simulink model "PNG3"  (R2021b)
settings: Solver=VariableStepAuto  StartTime=0.0  StopTime=45  RelTol=1e-3
values from neighbouring files (symbols this model uses):
  d2r = pi/180    (= 0.0174532925199)    [PN_Guidance_matlab.m]
  Ka = 4.5    [PN_Guidance_matlab.m]
  Kdc = 1.12    [PN_Guidance_matlab.m]
  Ki = 14.3    [PN_Guidance_matlab.m]
  Kr = -0.37    [PN_Guidance_matlab.m]
  l_M0 = 80*d2r    (= 1.3962634016)    [PN_Guidance_matlab.m]
  l_T0 = -2.5*d2r    (= -0.0436332312999)    [PN_Guidance_matlab.m]
  V_T = 600    [PN_Guidance_matlab.m]
  X_M0 = 2000    [PN_Guidance_matlab.m]
  X_T0 = 100    [PN_Guidance_matlab.m]
  Z_M0 = 0    [PN_Guidance_matlab.m]
  Z_T0 = 20000    [PN_Guidance_matlab.m]
libraries: simulink x1
settings Model: Creator=rocke  LastModifiedBy=rocke
settings SolverCC: ZeroCrossAlgorithm=Adaptive
settings DebuggingCC: IgnoredZcDiagnostic=none
settings SFSimCC: LegacyBehaviorForPersistentVarInContinuousTime=on

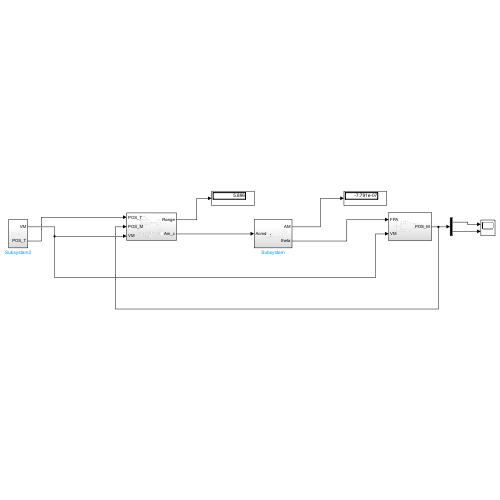
[thumbnail: Simulink's stored preview of the top-level diagram]
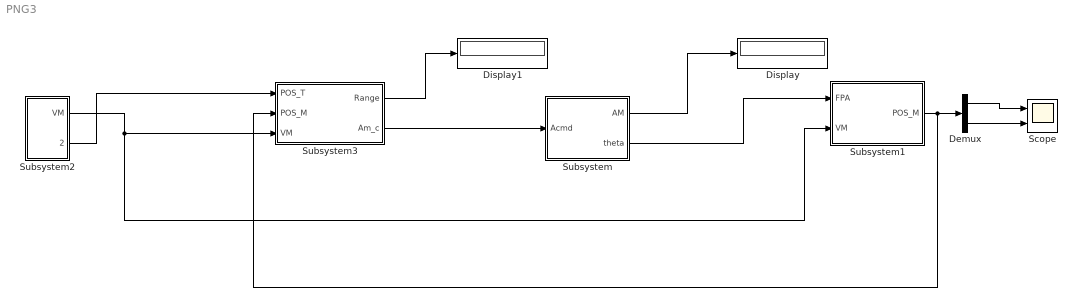
== system PNG3 ==
  Demux : Demux  Outputs=2
  Display : Display
  Display1 : Display
  Scope : Scope  NumInputPorts=2
  Subsystem : Subsystem
  Subsystem1 : Subsystem
  Subsystem2 : Subsystem
  Subsystem3 : Subsystem
  wires:
  Subsystem1/1(POS_M) -> Subsystem3/2(POS_M), Demux/1
  Demux/1 -> Scope/1
  Subsystem2/1(VM) -> Subsystem3/3(VM), Subsystem1/2(VM)
  Subsystem2/2(POS_T) -> Subsystem3/1(POS_T)
  Demux/2 -> Scope/2
  Subsystem3/1(Range) -> Display1/1
  Subsystem3/2(Am_c) -> Subsystem/1(Acmd)
  Subsystem/1(AM) -> Display/1
  Subsystem/2(theta) -> Subsystem1/1(FPA)

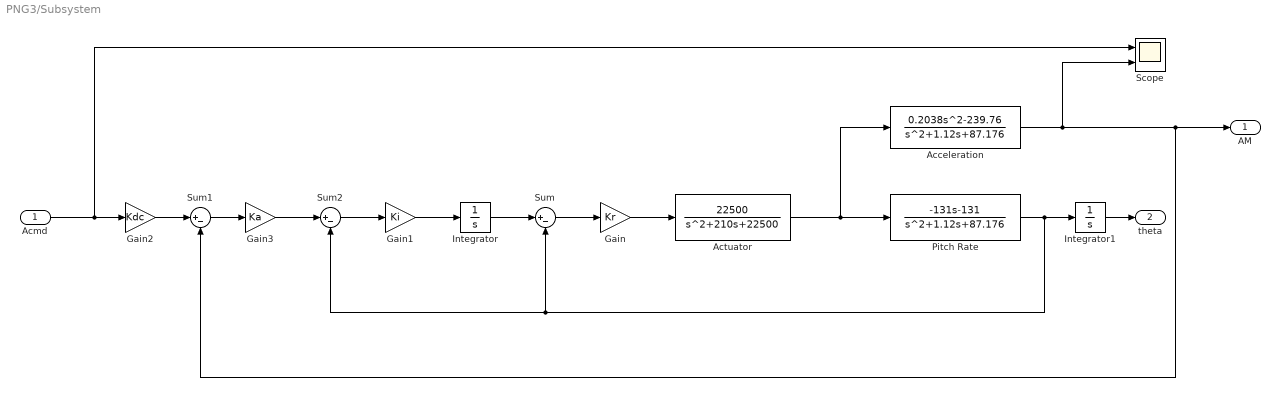
== system PNG3/Subsystem ==
  Acmd : Inport
  Acceleration : TransferFcn  Numerator=[0.2038 0 -239.76]  Denominator=[1 1.12 87.176]
  Actuator : TransferFcn  Numerator=[22500]  Denominator=[1 210 22500]
  Gain : Gain  Gain=Kr
  Gain1 : Gain  Gain=Ki
  Gain2 : Gain  Gain=Kdc
  Gain3 : Gain  Gain=Ka
  Integrator : Integrator
  Integrator1 : Integrator  InitialCondition=l_M0
  Pitch Rate : TransferFcn  Numerator=[-131 -131]  Denominator=[1 1.12 87.176]
  Scope : Scope  NumInputPorts=2
  Sum : Sum  Inputs=|+-
  Sum1 : Sum  Inputs=|+-
  Sum2 : Sum  Inputs=|+-
  AM : Outport
  theta : Outport  Port=2
  wires:
  Sum2/1 -> Gain1/1
  Gain3/1 -> Sum2/1
  Sum1/1 -> Gain3/1
  Gain2/1 -> Sum1/1
  Integrator/1 -> Sum/1
  Sum/1 -> Gain/1
  Gain1/1 -> Integrator/1
  Actuator/1 -> Acceleration/1, Pitch Rate/1
  Acceleration/1 -> Scope/2, AM/1, Sum1/2
  Integrator1/1 -> theta/1
  Acmd/1 -> Scope/1, Gain2/1
  Gain/1 -> Actuator/1
  Pitch Rate/1 -> Integrator1/1, Sum/2, Sum2/2

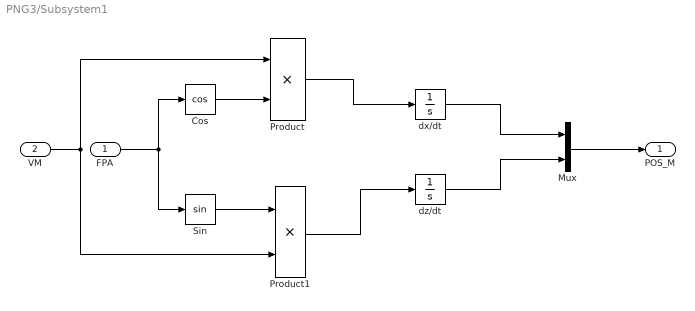
== system PNG3/Subsystem1 ==
  FPA : Inport
  VM : Inport  Port=2
  Cos : Trigonometry  Operator=cos
  Mux : Mux  Inputs=2
  Product : Product
  Product1 : Product
  Sin : Trigonometry
  dx/dt : Integrator  InitialCondition=X_M0
  dz/dt : Integrator  InitialCondition=Z_M0
  POS_M : Outport
  wires:
  Mux/1 -> POS_M/1
  dz/dt/1 -> Mux/2
  dx/dt/1 -> Mux/1
  VM/1 -> Product/1, Product1/2
  FPA/1 -> Sin/1, Cos/1
  Product/1 -> dx/dt/1
  Cos/1 -> Product/2
  Product1/1 -> dz/dt/1
  Sin/1 -> Product1/1

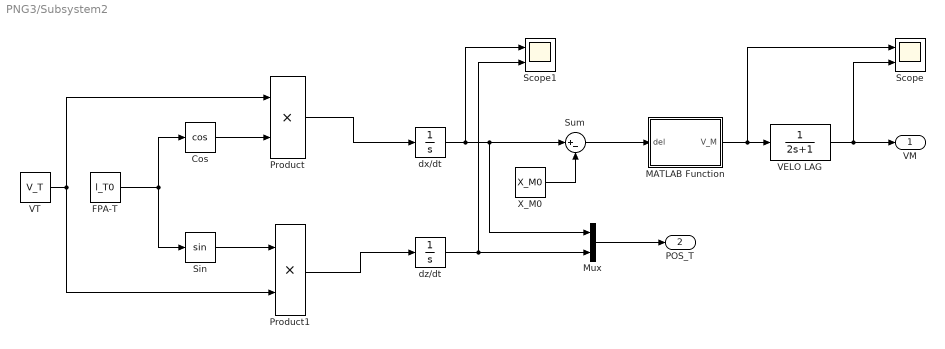
== system PNG3/Subsystem2 ==
  Cos : Trigonometry  Operator=cos
  FPA-T : Constant  Value=l_T0
  MATLAB Function : MATLAB Function  TreatAsAtomicUnit=on
  Mux : Mux  Inputs=2
  Product : Product
  Product1 : Product
  Scope : Scope  NumInputPorts=2
  Scope1 : Scope  NumInputPorts=2
  Sin : Trigonometry
  Sum : Sum  Inputs=|+-
  VELO LAG : TransferFcn  Denominator=[2 1]
  VT : Constant  Value=V_T
  X_M0 : Constant  Value=X_M0
  dx/dt : Integrator  InitialCondition=X_T0
  dz/dt : Integrator  InitialCondition=Z_T0
  VM : Outport
  POS_T : Outport  Port=2
  wires:
  VT/1 -> Product/1, Product1/2
  MATLAB Function/1(V_M) -> Scope/1, VELO LAG/1
  Cos/1 -> Product/2
  dx/dt/1 -> Scope1/1, Mux/1, Sum/1
  Mux/1 -> POS_T/1
  VELO LAG/1 -> VM/1, Scope/2
  Product/1 -> dx/dt/1
  dz/dt/1 -> Scope1/2, Mux/2
  X_M0/1 -> Sum/2
  FPA-T/1 -> Sin/1, Cos/1
  Sin/1 -> Product1/1
  Sum/1 -> MATLAB Function/1(del)
  Product1/1 -> dz/dt/1

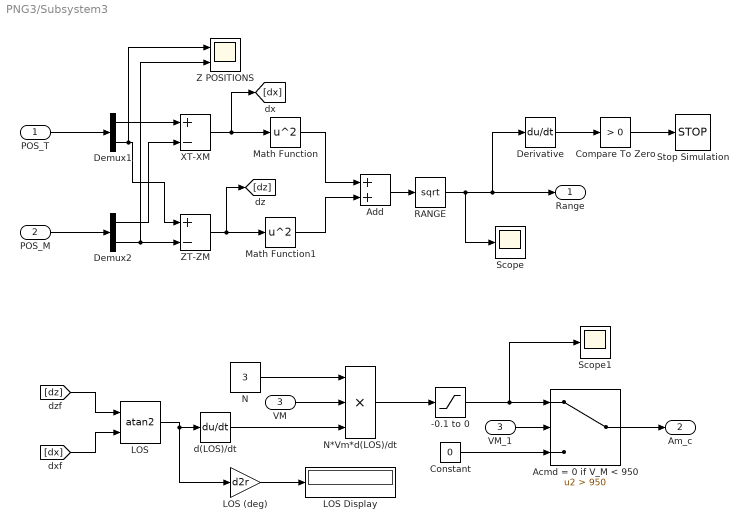
== system PNG3/Subsystem3 ==
  POS_T : Inport
  POS_M : Inport  Port=2
  VM : Inport  Port=3
  -0.1 to 0 : Saturate  UpperLimit=0  LowerLimit=-0.1
  Acmd = 0 if V_M < 950 : Switch  Criteria=u2 > Threshold  Threshold=950
  Add : Sum
  Compare To Zero : simulink/Logic and Bit Operations/Compare To Zero  relop=>  OutDataTypeStr=boolean
  Constant : Constant  Value=0
  Demux1 : Demux  Outputs=2
  Demux2 : Demux  Outputs=2
  Derivative : Derivative
  LOS : Trigonometry  Operator=atan2
  LOS (deg) : Gain  Gain=d2r
  LOS Display : Display
  Math Function : Math  Operator=square  SaturateOnIntegerOverflow=on
  Math Function1 : Math  Operator=square  SaturateOnIntegerOverflow=on
  N : Constant  Value=3
  N*Vm*d(LOS)/dt : Product  Inputs=3
  RANGE : Sqrt  SaturateOnIntegerOverflow=on
  Scope : Scope
  Scope1 : Scope
  Stop Simulation : Stop
  VM_1 : InportShadow  Port=3
  XT-XM : Sum  Inputs=+-
  Z POSITIONS : Scope  NumInputPorts=2
  ZT-ZM : Sum  Inputs=+-
  d(LOS)/dt : Derivative
  Range : Outport
  Am_c : Outport  Port=2
  wires:
  POS_M/1 -> Demux2/1
  POS_T/1 -> Demux1/1
  Math Function/1 -> Add/1
  Demux1/1 -> XT-XM/1
  ZT-ZM/1 -> [dz], Math Function1/1
  Derivative/1 -> Compare To Zero/1
  Demux2/1 -> XT-XM/2
  Demux2/2 -> Z POSITIONS/2, ZT-ZM/2
  Demux1/2 -> Z POSITIONS/1, ZT-ZM/1
  RANGE/1 -> Scope/1, Range/1, Derivative/1
  Add/1 -> RANGE/1
  XT-XM/1 -> [dx], Math Function/1
  Compare To Zero/1 -> Stop Simulation/1
  Math Function1/1 -> Add/2
  d(LOS)/dt/1 -> N*Vm*d(LOS)/dt/3
  LOS (deg)/1 -> LOS Display/1
  N*Vm*d(LOS)/dt/1 -> -0.1 to 0/1
  LOS/1 -> LOS (deg)/1, d(LOS)/dt/1
  VM_1/1 -> Acmd = 0 if V_M < 950/2
  -0.1 to 0/1 -> Scope1/1, Acmd = 0 if V_M < 950/1
  [dx] -> LOS/2
  Acmd = 0 if V_M < 950/1 -> Am_c/1
  [dz] -> LOS/1
  N/1 -> N*Vm*d(LOS)/dt/1
  VM/1 -> N*Vm*d(LOS)/dt/2
  Constant/1 -> Acmd = 0 if V_M < 950/3

== matlab function PNG3/Subsystem2/MATLAB Function ==
  data: del input; V_M output
function V_M = fcn(del)
%#codegen

persistent f 
persistent Vel

if isempty(f)
    f=0;
end
if isempty(Vel)
    Vel=0;
end

if f==0 && del > -200
    f=1;
    Vel=1021;
end

V_M=Vel;
